simulink model "step_response_rlc"  (R2016a)
settings: Solver=VariableStepAuto  StartTime=0.0  StopTime=0.001  RelTol=1e-3
settings Model: Creator=rashad  LastModifiedBy=rashad

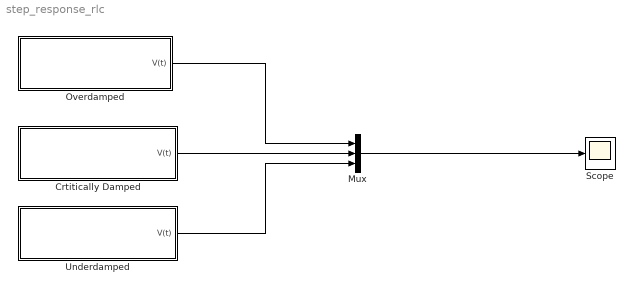
== system step_response_rlc ==
  "Crtitically Damped " : Subsystem
  Mux : Mux  Inputs=3
  "Overdamped " : Subsystem
  Scope : Scope
  "Underdamped " : Subsystem
  wires:
  "Underdamped "/1(V(t)) -> Mux/3
  Mux/1 -> Scope/1
  "Crtitically Damped "/1(V(t)) -> Mux/2
  "Overdamped "/1(V(t)) -> Mux/1

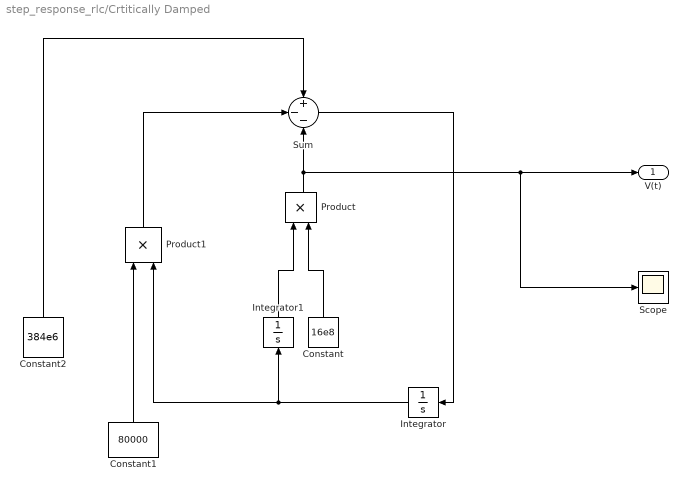
== system step_response_rlc/Crtitically Damped  ==
  Constant : Constant  Value=16e8
  Constant1 : Constant  Value=80000
  Constant2 : Constant  Value=384e6
  Integrator : Integrator
  Integrator1 : Integrator
  Product : Product
  Product1 : Product
  Scope : Scope
  Sum : Sum  Inputs=+--
  V(t) : Outport
  wires:
  Product1/1 -> Sum/2
  Constant1/1 -> Product1/1
  Constant/1 -> Product/2
  Constant2/1 -> Sum/1
  Product/1 -> Scope/1, V(t)/1, Sum/3
  Sum/1 -> Integrator/1
  Integrator/1 -> Product1/2, Integrator1/1
  Integrator1/1 -> Product/1

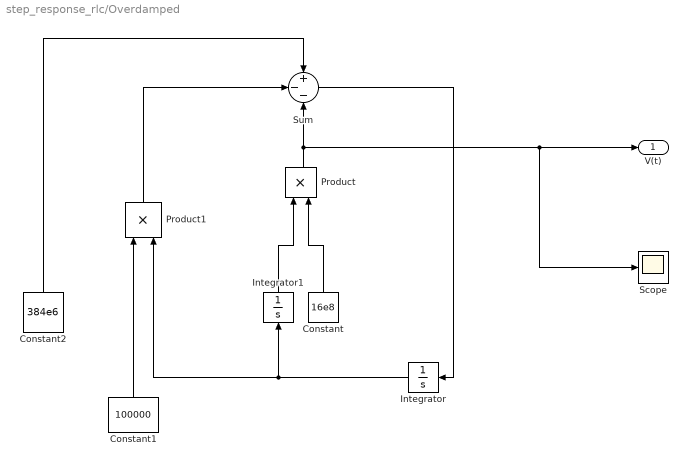
== system step_response_rlc/Overdamped  ==
  Constant : Constant  Value=16e8
  Constant1 : Constant  Value=100000
  Constant2 : Constant  Value=384e6
  Integrator : Integrator
  Integrator1 : Integrator
  Product : Product
  Product1 : Product
  Scope : Scope
  Sum : Sum  Inputs=+--
  V(t) : Outport
  wires:
  Product1/1 -> Sum/2
  Constant1/1 -> Product1/1
  Constant/1 -> Product/2
  Constant2/1 -> Sum/1
  Sum/1 -> Integrator/1
  Integrator/1 -> Product1/2, Integrator1/1
  Integrator1/1 -> Product/1
  Product/1 -> Scope/1, V(t)/1, Sum/3

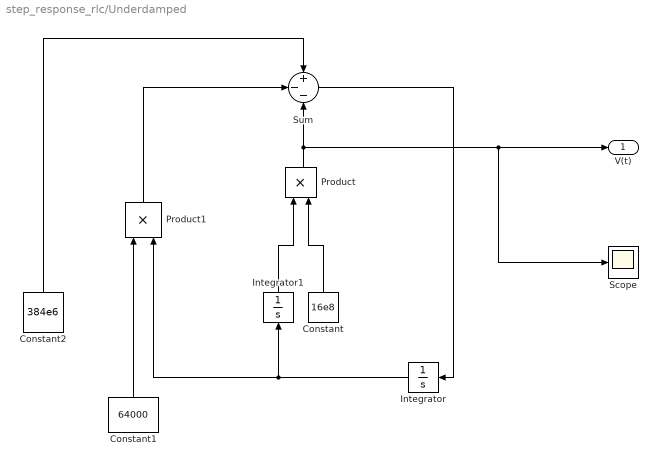
== system step_response_rlc/Underdamped  ==
  Constant : Constant  Value=16e8
  Constant1 : Constant  Value=64000
  Constant2 : Constant  Value=384e6
  Integrator : Integrator
  Integrator1 : Integrator
  Product : Product
  Product1 : Product
  Scope : Scope
  Sum : Sum  Inputs=+--
  V(t) : Outport
  wires:
  Sum/1 -> Integrator/1
  Integrator/1 -> Product1/2, Integrator1/1
  Constant/1 -> Product/2
  Integrator1/1 -> Product/1
  Product1/1 -> Sum/2
  Constant2/1 -> Sum/1
  Constant1/1 -> Product1/1
  Product/1 -> Scope/1, V(t)/1, Sum/3
